simulink model "lab1_PositionPIDController_Feedforward"  (R2020b)
settings: Solver=VariableStepAuto  StartTime=0.0  StopTime=20  RelTol=1e-3
undefined symbols (not defined in the file): Beq_hat, gbox, J_eq, K_D, k_drv, K_I, K_P, mot, R_eq, rpm2rads, sens, T_L, tau_sf_hat
libraries: simulink x1
settings Model: Creator=Musta  LastModifiedBy=Musta

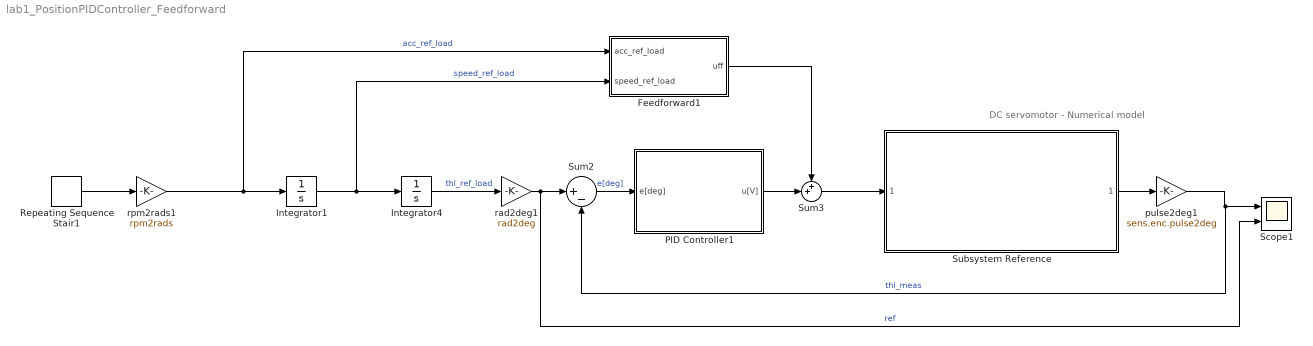
== system lab1_PositionPIDController_Feedforward ==
  note: DC servomotor - Numerical model
  Feedforward1 : Subsystem
  Integrator1 : Integrator
  Integrator4 : Integrator
  PID Controller1 : Subsystem
  Repeating Sequence Stair1 : simulink/Sources/Repeating Sequence Stair  OutValues=[900 0 -900 -900 0 900]  tsamp=0.5  OutMin=[]  OutMax=[]  OutDataTypeStr=double  OutputDataTypeScalingMode=double  OutDataType=fixdt(0,8)  ConRadixGroup=Best Precision: Vector-wise  OutScaling=2^-12
  Scope1 : Scope  NumInputPorts=2
  Subsystem Reference : Subsystem  ReferencedSubsystem=plant_Model
  Sum2 : Sum  Inputs=|+-
  Sum3 : Sum  Inputs=++|
  pulse2deg1 : Gain  Gain=sens.enc.pulse2deg
  rad2deg1 : Gain  Gain=rad2deg
  rpm2rads1 : Gain  Gain=rpm2rads
  wires:
  rad2deg1/1 -> Scope1/2, Sum2/1  "ref"
  Feedforward1/1(uff) -> Sum3/1
  Integrator4/1 -> rad2deg1/1  "thl_ref_load"
  Sum2/1 -> PID Controller1/1(e[deg])  "e[deg]"
  Repeating Sequence Stair1/1 -> rpm2rads1/1
  rpm2rads1/1 -> Feedforward1/1(acc_ref_load), Integrator1/1  "acc_ref_load"
  PID Controller1/1(u[V]) -> Sum3/2
  Integrator1/1 -> Integrator4/1, Feedforward1/2(speed_ref_load)  "speed_ref_load"
  Sum3/1 -> Subsystem Reference/1
  pulse2deg1/1 -> Sum2/2, Scope1/1  "thi_meas"
  Subsystem Reference/1 -> pulse2deg1/1

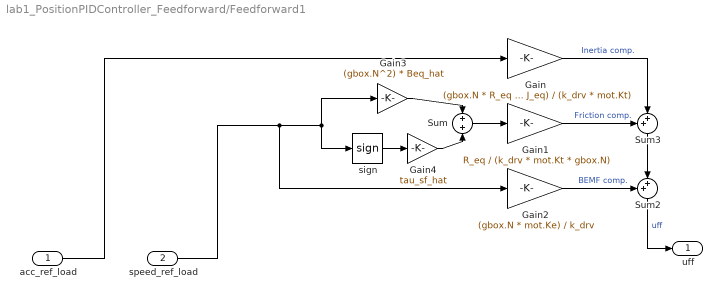
== system lab1_PositionPIDController_Feedforward/Feedforward1 ==
  acc_ref_load : Inport
  speed_ref_load : Inport  Port=2
  Gain : Gain  Gain=(gbox.N * R_eq * J_eq) / (k_drv * mot.Kt)
  Gain1 : Gain  Gain=R_eq / (k_drv * mot.Kt * gbox.N)
  Gain2 : Gain  Gain=(gbox.N * mot.Ke) / k_drv
  Gain3 : Gain  Gain=(gbox.N^2) * Beq_hat
  Gain4 : Gain  Gain=tau_sf_hat
  Sum : Sum  Inputs=+|+
  Sum2 : Sum  Inputs=++|
  Sum3 : Sum  Inputs=++|
  sign : Signum
  uff : Outport
  wires:
  sign/1 -> Gain4/1
  Sum/1 -> Gain1/1
  speed_ref_load/1 -> Gain2/1, sign/1, Gain3/1
  Sum3/1 -> Sum2/2
  Gain3/1 -> Sum/1
  Gain/1 -> Sum3/2  "Inertia comp."
  Gain1/1 -> Sum3/1  "Friction comp."
  Gain4/1 -> Sum/2
  Gain2/1 -> Sum2/1  "BEMF comp."
  acc_ref_load/1 -> Gain/1
  Sum2/1 -> uff/1  "uff"

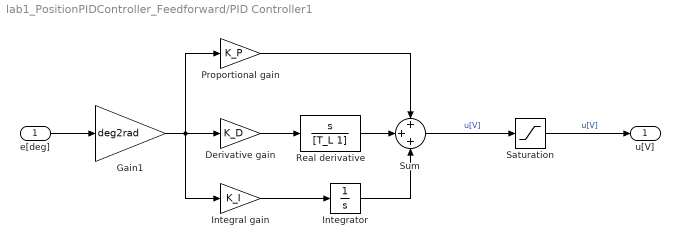
== system lab1_PositionPIDController_Feedforward/PID Controller1 ==
  e[deg] : Inport
  Derivative gain : Gain  Gain=K_D
  Gain1 : Gain  Gain=deg2rad
  Integral gain : Gain  Gain=K_I
  Integrator : Integrator
  Proportional gain : Gain  Gain=K_P
  Real derivative : TransferFcn  Numerator=[1 0]  Denominator=[T_L 1]
  Saturation : Saturate  UpperLimit=10  LowerLimit=-10
  Sum : Sum  Inputs=+++
  u[V] : Outport
  wires:
  e[deg]/1 -> Gain1/1
  Real derivative/1 -> Sum/2
  Gain1/1 -> Derivative gain/1, Integral gain/1, Proportional gain/1
  Proportional gain/1 -> Sum/1
  Integrator/1 -> Sum/3
  Derivative gain/1 -> Real derivative/1
  Sum/1 -> Saturation/1  "u[V]"
  Saturation/1 -> u[V]/1  "u[V]"
  Integral gain/1 -> Integrator/1
